simulink model "sysID_1"  (R2024a)
settings: Solver=VariableStepAuto  StartTime=0.0  StopTime=T  RelTol=1e-3
values from neighbouring files (symbols this model uses):
  T = 10    [systemID.m]    (also in systemID_initialization.m = 15)
  Ts = 1    [systemID.m]    (also in systemID_initialization.m = 0.002)
settings Model: Creator=dunni  LastModifiedBy=dunni

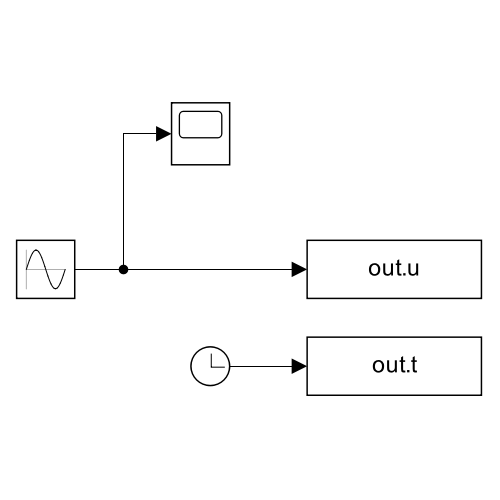
[thumbnail: Simulink's stored preview of the top-level diagram]
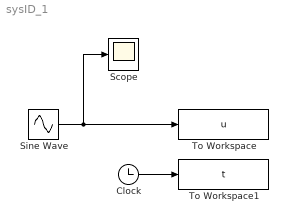
== system sysID_1 ==
  Clock : Clock
  Scope : Scope
  Sine Wave : Sin  Frequency=2*pi/T  SampleTime=0
  To Workspace : ToWorkspace  VariableName=u  SampleTime=Ts
  To Workspace1 : ToWorkspace  VariableName=t  SampleTime=Ts
  wires:
  Sine Wave/1 -> To Workspace/1, Scope/1
  Clock/1 -> To Workspace1/1
